simulink model "robot_step"  (Simulink 7.4)
settings: Solver=FixedStepDiscrete  StartTime=0.0  StopTime=50  FixedStep=0.1  RelTol=1e-3
values from neighbouring files (symbols this model uses):
  Link1 = [pi/2, 0, pi/2, 0]    [robot_parameters.m]
  Link2 = [0, 0.404, pi/2, 0]    [robot_parameters.m]
  Link3 = [-pi/2, 0, 0, 0]    [robot_parameters.m]
  Link4 = [pi/2, 0.025, 0, 0.405]    [robot_parameters.m]
  Link5 = [pi/2, 0, pi/2, 0]    [robot_parameters.m]
  Link6 = [0, 0, pi/2, 0]    [robot_parameters.m]
  NoOfLinks = 6    [robot_parameters.m]
libraries: vrlib x3, simulink x2
settings Model: Creator=angelosanto  LastModifiedBy=indranilsaha  BufferReuse=off
settings OptimizationCC: BlockReduction=off  BooleanDataType=off  ConditionallyExecuteInputs=off  InlineParams=on  OptimizeBlockIOStorage=off  BufferReuse=off  ExpressionFolding=off  LocalBlockOutputs=off
settings RTWCC: GenCodeOnly=on  GenerateMakefile=off

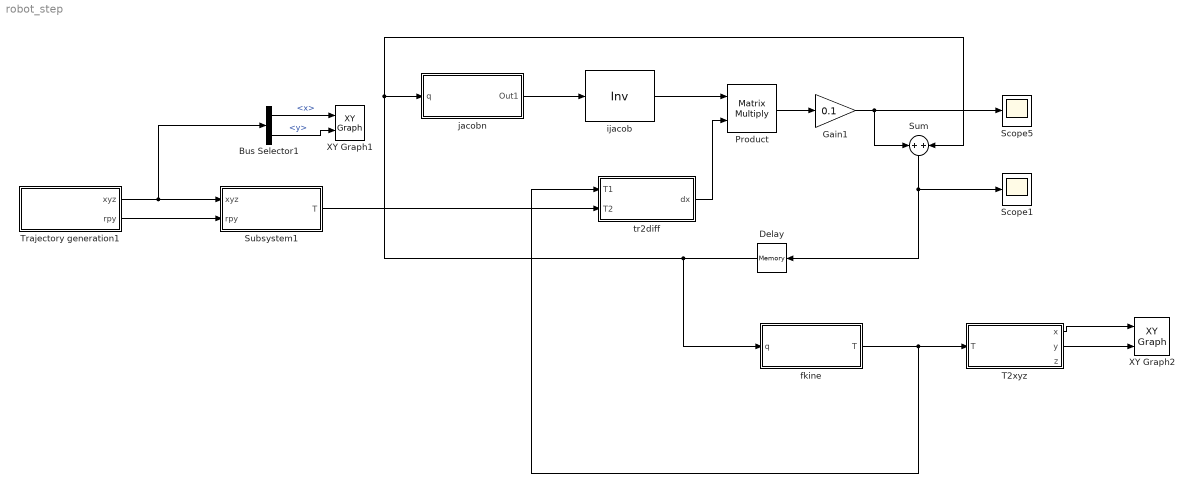
== system robot_step ==
  Bus Selector1 : BusSelector  OutputSignals=x,y
  Delay : Memory  X0=[pi/2; pi/2; 0; 0; pi/2; pi/2]  InheritSampleTime=on
  Gain1 : Gain  Gain=0.1  ParameterDataType=fixdt(1, 16)  ParameterScaling=2^0  OutDataType=fixdt(1, 16)  OutScaling=2^0
  Product : Product  Multiplication=Matrix(*)  OutDataType=sfix(16)  OutScaling=2^0  RndMeth=Zero
  Scope1 : Scope
      settings: YMin=-1  YMax=4
  Scope5 : Scope
      settings: YMin=-0.0003  YMax=0.00025  SaveName=ScopeData3
  Subsystem1 : Subsystem
  Sum : Sum  OutDataType=sfix(16)  OutScaling=2^0
  T2xyz : Subsystem
  Trajectory generation1 : Subsystem
  XY Graph1 : simulink/Sinks/XY Graph  SystemSampleTime=-1  xmin=-1.5  xmax=1.5  ymin=-1.5  ymax=1.5  st=-1
  XY Graph2 : simulink/Sinks/XY Graph  SystemSampleTime=-1  xmin=-1.5  xmax=1.5  ymin=-1.5  ymax=1.5  st=-1
  fkine : Subsystem  TreatAsAtomicUnit=on
  ijacob : Product  Inputs=/  Multiplication=Matrix(*)  OutDataType=fixdt(1, 16)  OutScaling=2^0  RndMeth=Zero
  jacobn : Subsystem  TreatAsAtomicUnit=on
  tr2diff : Subsystem
  wires:
  T2xyz/1(x) -> XY Graph2/1
  T2xyz/2(y) -> XY Graph2/2
  fkine/1(T) -> T2xyz/1(T), tr2diff/1(T1)
  jacobn/1(Out1) -> ijacob/1
  ijacob/1 -> Product/1
  tr2diff/1(dx) -> Product/2
  Sum/1 -> Delay/1, Scope1/1
  Delay/1 -> Sum/2, jacobn/1(q), fkine/1(q)
  Trajectory generation1/1(xyz) -> Subsystem1/1(xyz), Bus Selector1/1
  Trajectory generation1/2(rpy) -> Subsystem1/2(rpy)
  Bus Selector1/1 -> XY Graph1/1  "<x>"
  Bus Selector1/2 -> XY Graph1/2  "<y>"
  Subsystem1/1(T) -> tr2diff/2(T2)
  Product/1 -> Gain1/1
  Gain1/1 -> Scope5/1, Sum/1

== system robot_step/Subsystem1 ==
  xyz : Inport  OutDataType=fixdt(1, 16)  OutScaling=2^0
  rpy : Inport  Port=2  OutDataType=fixdt(1, 16)  OutScaling=2^0
  Bus Selector : BusSelector  OutputSignals=x,y,z
  Bus Selector1 : BusSelector  OutputSignals=roll,pitch,yaw
  Product : Product  Multiplication=Matrix(*)  OutDataType=fixdt(1, 16)  OutScaling=2^0  RndMeth=Zero
  rpy2T : Subsystem
  xyz2T : Subsystem
  T : Outport  OutDataType=fixdt(1, 16)  OutScaling=2^0
  wires:
  xyz/1 -> Bus Selector/1
  Bus Selector/1 -> xyz2T/1(x)  "<x>"
  Bus Selector/2 -> xyz2T/2(y)  "<y>"
  Bus Selector/3 -> xyz2T/3(z)  "<z>"
  xyz2T/1(T) -> Product/1
  Product/1 -> T/1
  rpy2T/1(T) -> Product/2
  rpy/1 -> Bus Selector1/1
  Bus Selector1/1 -> rpy2T/1(roll)  "<roll>"
  Bus Selector1/2 -> rpy2T/2(pitch)  "<pitch>"
  Bus Selector1/3 -> rpy2T/3(yaw)  "<yaw>"

== system robot_step/T2xyz ==
  T : Inport  OutDataType=fixdt(1, 16)  OutScaling=2^0
  Selector : Selector  NumberOfDimensions=2  InputPortWidth=3  IndexOptions=Index vector (dialog),Index vector (dialog)  Indices=1,4  OutputSizes=1,1
  Selector1 : Selector  NumberOfDimensions=2  InputPortWidth=3  IndexOptions=Index vector (dialog),Index vector (dialog)  Indices=2,4  OutputSizes=1,1
  Selector2 : Selector  NumberOfDimensions=2  InputPortWidth=3  IndexOptions=Index vector (dialog),Index vector (dialog)  Indices=3,4  OutputSizes=1,1
  x : Outport  OutDataType=fixdt(1, 16)  OutScaling=2^0
  y : Outport  Port=2  OutDataType=fixdt(1, 16)  OutScaling=2^0
  z : Outport  Port=3  OutDataType=fixdt(1, 16)  OutScaling=2^0
  wires:
  Selector/1 -> x/1
  Selector1/1 -> y/1
  Selector2/1 -> z/1
  T/1 -> Selector/1, Selector2/1, Selector1/1

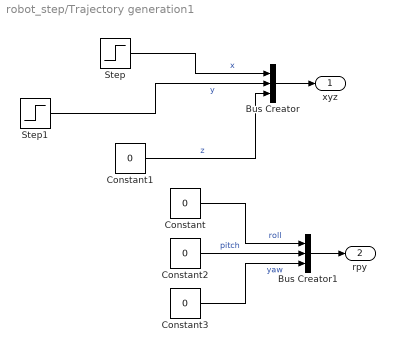
== system robot_step/Trajectory generation1 ==
  Bus Creator : BusCreator  Inputs=3
  Bus Creator1 : BusCreator  Inputs=3
  Constant : Constant  Value=0  VectorParams1D=off  OutDataType=fixdt(1, 16)  OutScaling=2^0
  Constant1 : Constant  Value=0
  Constant2 : Constant  Value=0  OutDataType=fixdt(1, 16)  OutScaling=2^0
  Constant3 : Constant  Value=0  OutDataType=fixdt(1, 16)  OutScaling=2^0
  Step : Step  After=0.3  SampleTime=0
  Step1 : Step  After=0.3  SampleTime=0
  xyz : Outport  OutDataType=fixdt(1, 16)  OutScaling=2^0
  rpy : Outport  Port=2  OutDataType=fixdt(1, 16)  OutScaling=2^0
  wires:
  Constant1/1 -> Bus Creator/3  "z"
  Bus Creator/1 -> xyz/1
  Constant2/1 -> Bus Creator1/2  "pitch"
  Constant/1 -> Bus Creator1/1  "roll"
  Constant3/1 -> Bus Creator1/3  "yaw"
  Bus Creator1/1 -> rpy/1
  Step/1 -> Bus Creator/1  "x"
  Step1/1 -> Bus Creator/2  "y"

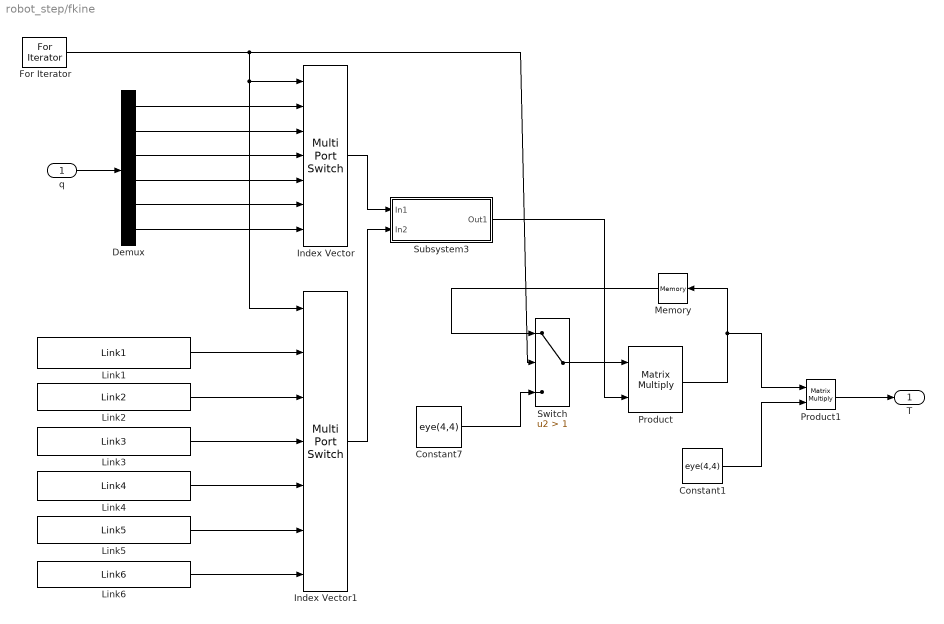
== system robot_step/fkine ==
  q : Inport  OutDataType=fixdt(1, 16)  OutScaling=2^0
  Constant1 : Constant  Value=eye(4,4)  OutDataType=fixdt(1, 16)  OutScaling=2^0
  Constant7 : Constant  Value=eye(4,4)  OutDataType=fixdt(1, 16)  OutScaling=2^0
  Demux : Demux  Outputs=6
  For Iterator : ForIterator  IterationLimit=NoOfLinks
  Index Vector : MultiPortSwitch  Inputs=6  OutDataType=fixdt(1, 16)  OutScaling=2^0
  Index Vector1 : MultiPortSwitch  Inputs=6  OutDataType=fixdt(1, 16)  OutScaling=2^0
  Link1 : Constant  Value=Link1  OutDataType=fixdt(1, 16)  OutScaling=2^0
  Link2 : Constant  Value=Link2  OutDataType=fixdt(1, 16)  OutScaling=2^0
  Link3 : Constant  Value=Link3  OutDataType=fixdt(1, 16)  OutScaling=2^0
  Link4 : Constant  Value=Link4  OutDataType=fixdt(1, 16)  OutScaling=2^0
  Link5 : Constant  Value=Link5  OutDataType=fixdt(1, 16)  OutScaling=2^0
  Link6 : Constant  Value=Link6  OutDataType=fixdt(1, 16)  OutScaling=2^0
  Memory : Memory  X0=eye(4,4)  InheritSampleTime=on
  Product : Product  Multiplication=Matrix(*)  OutDataType=fixdt(1, 16)  OutScaling=2^0  RndMeth=Zero
  Product1 : Product  Multiplication=Matrix(*)  OutDataType=fixdt(1, 16)  OutScaling=2^0  RndMeth=Zero
  Subsystem3 : Subsystem
  Switch : Switch  Criteria=u2 > Threshold  Threshold=1  OutDataType=fixdt(1, 16)  OutScaling=2^0
  T : Outport  OutDataType=fixdt(1, 16)  OutScaling=2^0
  wires:
  Memory/1 -> Switch/1
  Switch/1 -> Product/1
  Subsystem3/1(Out1) -> Product/2
  Constant7/1 -> Switch/3
  Product/1 -> Product1/1, Memory/1
  Index Vector1/1 -> Subsystem3/2(In2)
  Index Vector/1 -> Subsystem3/1(In1)
  Demux/6 -> Index Vector/7
  Demux/5 -> Index Vector/6
  Demux/4 -> Index Vector/5
  Demux/3 -> Index Vector/4
  Demux/2 -> Index Vector/3
  Demux/1 -> Index Vector/2
  q/1 -> Demux/1
  Link6/1 -> Index Vector1/7
  Link5/1 -> Index Vector1/6
  Link4/1 -> Index Vector1/5
  Link3/1 -> Index Vector1/4
  Link2/1 -> Index Vector1/3
  Link1/1 -> Index Vector1/2
  For Iterator/1 -> Switch/2, Index Vector1/1, Index Vector/1
  Product1/1 -> T/1
  Constant1/1 -> Product1/2

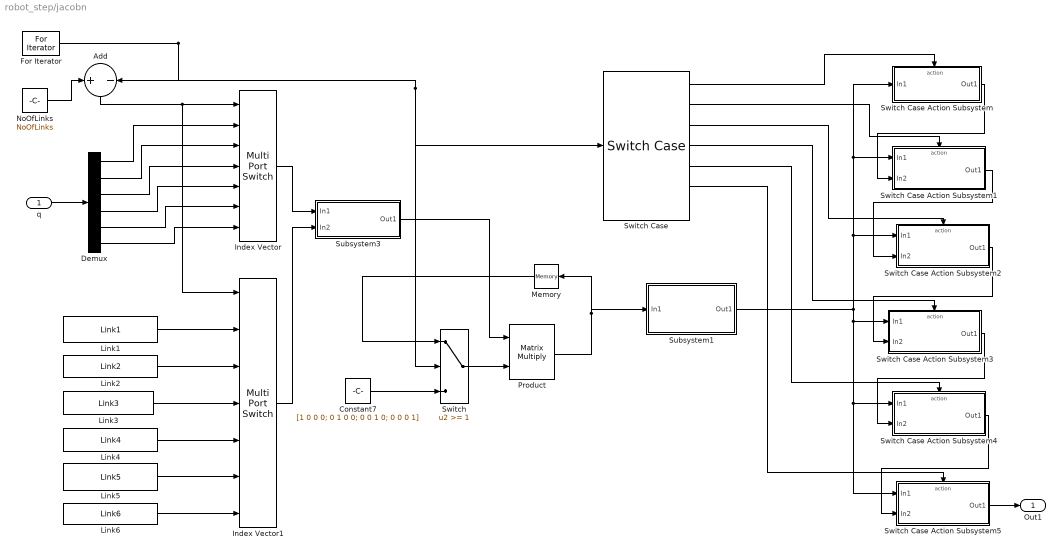
== system robot_step/jacobn ==
  q : Inport  OutDataType=fixdt(1, 16)  OutScaling=2^0
  Add : Sum  Inputs=+-  OutDataType=fixdt(1, 16)  OutScaling=2^-10
  Constant7 : Constant  Value=[1 0 0 0; 0 1 0 0; 0 0 1 0; 0 0 0 1]  OutDataType=fixdt(1, 16)  OutScaling=2^0
  Demux : Demux  Outputs=6
  For Iterator : ForIterator  IterationLimit=NoOfLinks
  Index Vector : MultiPortSwitch  Inputs=6  zeroidx=on  OutDataType=fixdt(1, 16)  OutScaling=2^0
  Index Vector1 : MultiPortSwitch  Inputs=6  zeroidx=on  OutDataType=fixdt(1, 16)  OutScaling=2^0
  Link1 : Constant  Value=Link1  OutDataType=fixdt(1, 16)  OutScaling=2^0
  Link2 : Constant  Value=Link2  OutDataType=fixdt(1, 16)  OutScaling=2^0
  Link3 : Constant  Value=Link3  OutDataType=fixdt(1, 16)  OutScaling=2^0
  Link4 : Constant  Value=Link4  OutDataType=fixdt(1, 16)  OutScaling=2^0
  Link5 : Constant  Value=Link5  OutDataType=fixdt(1, 16)  OutScaling=2^0
  Link6 : Constant  Value=Link6  OutDataType=fixdt(1, 16)  OutScaling=2^0
  Memory : Memory  X0=[1 0 0 0; 0 1 0 0; 0 0 1 0; 0 0 0 1]  InheritSampleTime=on
  NoOfLinks : Constant  Value=NoOfLinks  OutDataType=fixdt(1, 16)  OutScaling=2^0
  Product : Product  Multiplication=Matrix(*)  OutDataType=fixdt(1, 16)  OutScaling=2^0  RndMeth=Zero
  Subsystem1 : Subsystem
  Subsystem3 : Subsystem
  Switch : Switch  Threshold=1  OutDataType=fixdt(1, 16)  OutScaling=2^0
  Switch Case : SwitchCase  CaseConditions={1, 2, 3, 4, 5, 6}
  Switch Case Action Subsystem : Subsystem  TreatAsAtomicUnit=on
  Switch Case Action Subsystem1 : Subsystem  TreatAsAtomicUnit=on
  Switch Case Action Subsystem2 : Subsystem  TreatAsAtomicUnit=on
  Switch Case Action Subsystem3 : Subsystem  TreatAsAtomicUnit=on
  Switch Case Action Subsystem4 : Subsystem  TreatAsAtomicUnit=on
  Switch Case Action Subsystem5 : Subsystem  TreatAsAtomicUnit=on
  Out1 : Outport  OutDataType=fixdt(1, 16)  OutScaling=2^0
  wires:
  NoOfLinks/1 -> Add/1
  For Iterator/1 -> Add/2, Switch/2, Switch Case/1
  Add/1 -> Index Vector/1, Index Vector1/1
  Link1/1 -> Index Vector1/2
  Link2/1 -> Index Vector1/3
  Link3/1 -> Index Vector1/4
  Link4/1 -> Index Vector1/5
  Link5/1 -> Index Vector1/6
  Link6/1 -> Index Vector1/7
  q/1 -> Demux/1
  Demux/1 -> Index Vector/2
  Demux/2 -> Index Vector/3
  Demux/3 -> Index Vector/4
  Demux/4 -> Index Vector/5
  Demux/5 -> Index Vector/6
  Demux/6 -> Index Vector/7
  Index Vector/1 -> Subsystem3/1(In1)
  Index Vector1/1 -> Subsystem3/2(In2)
  Product/1 -> Memory/1, Subsystem1/1(In1)
  Constant7/1 -> Switch/3
  Subsystem3/1(Out1) -> Product/1
  Switch/1 -> Product/2
  Memory/1 -> Switch/1
  Subsystem1/1(Out1) -> Switch Case Action Subsystem/1(In1), Switch Case Action Subsystem1/1(In1), Switch Case Action Subsystem2/1(In1), Switch Case Action Subsystem5/1(In1), Switch Case Action Subsystem4/1(In1), Switch Case Action Subsystem3/1(In1)
  Switch Case/1 -> Switch Case Action Subsystem/Action
  Switch Case/2 -> Switch Case Action Subsystem1/Action
  Switch Case/3 -> Switch Case Action Subsystem2/Action
  Switch Case/4 -> Switch Case Action Subsystem3/Action
  Switch Case/5 -> Switch Case Action Subsystem4/Action
  Switch Case/6 -> Switch Case Action Subsystem5/Action
  Switch Case Action Subsystem5/1(Out1) -> Out1/1
  Switch Case Action Subsystem1/1(Out1) -> Switch Case Action Subsystem2/2(In2)
  Switch Case Action Subsystem/1(Out1) -> Switch Case Action Subsystem1/2(In2)
  Switch Case Action Subsystem2/1(Out1) -> Switch Case Action Subsystem3/2(In2)
  Switch Case Action Subsystem3/1(Out1) -> Switch Case Action Subsystem4/2(In2)
  Switch Case Action Subsystem4/1(Out1) -> Switch Case Action Subsystem5/2(In2)

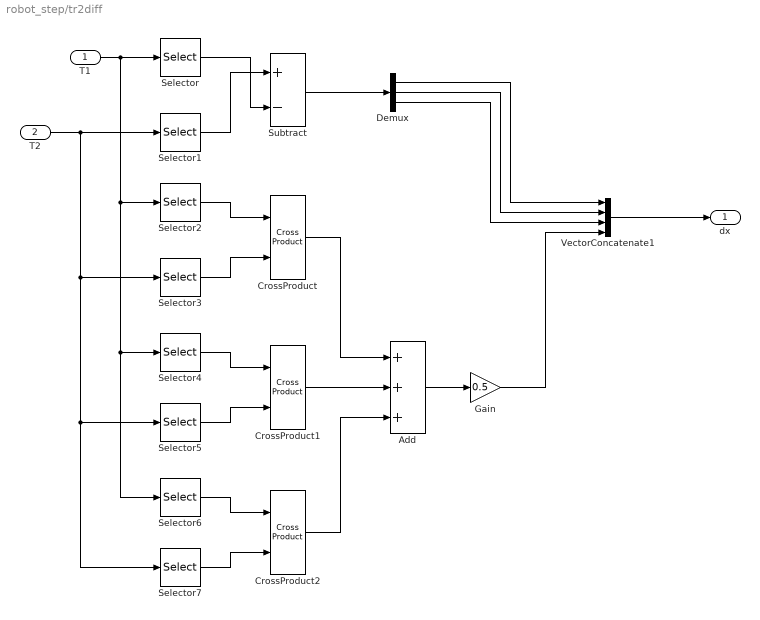
== system robot_step/tr2diff ==
  T1 : Inport  OutDataType=fixdt(1, 16)  OutScaling=2^0
  T2 : Inport  Port=2  OutDataType=fixdt(1, 16)  OutScaling=2^0
  Add : Sum  Inputs=+++  OutDataType=fixdt(1, 16)  OutScaling=2^-10
  CrossProduct : vrlib/Utilities/Cross Product  SystemSampleTime=-1
  CrossProduct1 : vrlib/Utilities/Cross Product  SystemSampleTime=-1
  CrossProduct2 : vrlib/Utilities/Cross Product  SystemSampleTime=-1
  Demux : Demux  Outputs=3
  Gain : Gain  Gain=0.5  ParameterDataType=fixdt(1, 16)  ParameterScaling=2^0  OutDataType=fixdt(1, 16)  OutScaling=2^0
  Selector : Selector  NumberOfDimensions=2  InputPortWidth=3  IndexOptions=Index vector (dialog),Index vector (dialog)  Indices=[1:3],4  OutputSizes=1,1
  Selector1 : Selector  NumberOfDimensions=2  InputPortWidth=3  IndexOptions=Index vector (dialog),Index vector (dialog)  Indices=[1:3],4  OutputSizes=1,1
  Selector2 : Selector  NumberOfDimensions=2  InputPortWidth=3  IndexOptions=Index vector (dialog),Index vector (dialog)  Indices=[1:3],1  OutputSizes=1,1
  Selector3 : Selector  NumberOfDimensions=2  InputPortWidth=3  IndexOptions=Index vector (dialog),Index vector (dialog)  Indices=[1:3],1  OutputSizes=1,1
  Selector4 : Selector  NumberOfDimensions=2  InputPortWidth=3  IndexOptions=Index vector (dialog),Index vector (dialog)  Indices=[1:3],2  OutputSizes=1,1
  Selector5 : Selector  NumberOfDimensions=2  InputPortWidth=3  IndexOptions=Index vector (dialog),Index vector (dialog)  Indices=[1:3],2  OutputSizes=1,1
  Selector6 : Selector  NumberOfDimensions=2  InputPortWidth=3  IndexOptions=Index vector (dialog),Index vector (dialog)  Indices=[1:3],3  OutputSizes=1,1
  Selector7 : Selector  NumberOfDimensions=2  InputPortWidth=3  IndexOptions=Index vector (dialog),Index vector (dialog)  Indices=[1:3],3  OutputSizes=1,1
  Subtract : Sum  Inputs=+-  OutDataType=fixdt(1, 16)  OutScaling=2^-10
  VectorConcatenate1 : Concatenate  NumInputs=4  Mode=Vector
  dx : Outport  OutDataType=fixdt(1, 16)  OutScaling=2^0
  wires:
  T1/1 -> Selector/1, Selector2/1, Selector6/1, Selector4/1
  T2/1 -> Selector1/1, Selector7/1, Selector5/1, Selector3/1
  Selector1/1 -> Subtract/1
  Selector/1 -> Subtract/2
  Selector2/1 -> CrossProduct/1
  Selector3/1 -> CrossProduct/2
  Selector4/1 -> CrossProduct1/1
  Selector5/1 -> CrossProduct1/2
  Selector6/1 -> CrossProduct2/1
  Selector7/1 -> CrossProduct2/2
  CrossProduct/1 -> Add/1
  CrossProduct1/1 -> Add/2
  CrossProduct2/1 -> Add/3
  Add/1 -> Gain/1
  VectorConcatenate1/1 -> dx/1
  Subtract/1 -> Demux/1
  Demux/1 -> VectorConcatenate1/1
  Demux/2 -> VectorConcatenate1/2
  Demux/3 -> VectorConcatenate1/3
  Gain/1 -> VectorConcatenate1/4

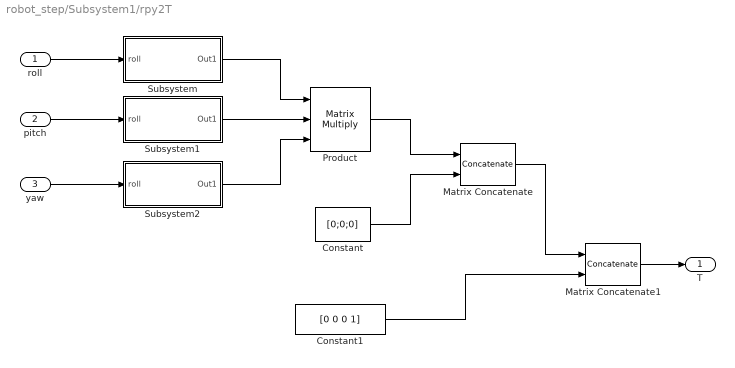
== system robot_step/Subsystem1/rpy2T ==
  roll : Inport  OutDataType=fixdt(1, 16)  OutScaling=2^0
  pitch : Inport  Port=2  OutDataType=fixdt(1, 16)  OutScaling=2^0
  yaw : Inport  Port=3  OutDataType=fixdt(1, 16)  OutScaling=2^0
  Constant : Constant  Value=[0;0;0]  OutDataType=fixdt(1, 16)  OutScaling=2^0
  Constant1 : Constant  Value=[0 0 0 1]  VectorParams1D=off  OutDataType=fixdt(1, 16)  OutScaling=2^0
  Matrix Concatenate : Concatenate  Mode=Multidimensional array  ConcatenateDimension=2
  Matrix Concatenate1 : Concatenate  Mode=Multidimensional array
  Product : Product  Inputs=3  Multiplication=Matrix(*)  OutDataType=fixdt(1, 16)  OutScaling=2^0  RndMeth=Zero
  Subsystem : Subsystem
  Subsystem1 : Subsystem
  Subsystem2 : Subsystem
  T : Outport  OutDataType=fixdt(1, 16)  OutScaling=2^0
  wires:
  roll/1 -> Subsystem/1(roll)
  pitch/1 -> Subsystem1/1(roll)
  yaw/1 -> Subsystem2/1(roll)
  Subsystem/1(Out1) -> Product/1
  Subsystem1/1(Out1) -> Product/2
  Subsystem2/1(Out1) -> Product/3
  Product/1 -> Matrix Concatenate/1
  Constant/1 -> Matrix Concatenate/2
  Matrix Concatenate/1 -> Matrix Concatenate1/1
  Constant1/1 -> Matrix Concatenate1/2
  Matrix Concatenate1/1 -> T/1

== system robot_step/Subsystem1/xyz2T ==
  x : Inport  OutDataType=fixdt(1, 16)  OutScaling=2^0
  y : Inport  Port=2  OutDataType=fixdt(1, 16)  OutScaling=2^0
  z : Inport  Port=3  OutDataType=fixdt(1, 16)  OutScaling=2^0
  Constant : Constant  Value=eye(3)  OutDataType=fixdt(1, 16)  OutScaling=2^0
  Constant1 : Constant  Value=[0 0 0 1]  VectorParams1D=off  OutDataType=fixdt(1, 16)  OutScaling=2^0
  Matrix Concatenate : Concatenate  Mode=Multidimensional array  ConcatenateDimension=2
  Matrix Concatenate1 : Concatenate  Mode=Multidimensional array
  Vector Concatenate : Concatenate  NumInputs=3  Mode=Vector
  T : Outport  OutDataType=fixdt(1, 16)  OutScaling=2^0
  wires:
  x/1 -> Vector Concatenate/1
  y/1 -> Vector Concatenate/2
  z/1 -> Vector Concatenate/3
  Constant/1 -> Matrix Concatenate/1
  Vector Concatenate/1 -> Matrix Concatenate/2
  Matrix Concatenate/1 -> Matrix Concatenate1/1
  Constant1/1 -> Matrix Concatenate1/2
  Matrix Concatenate1/1 -> T/1

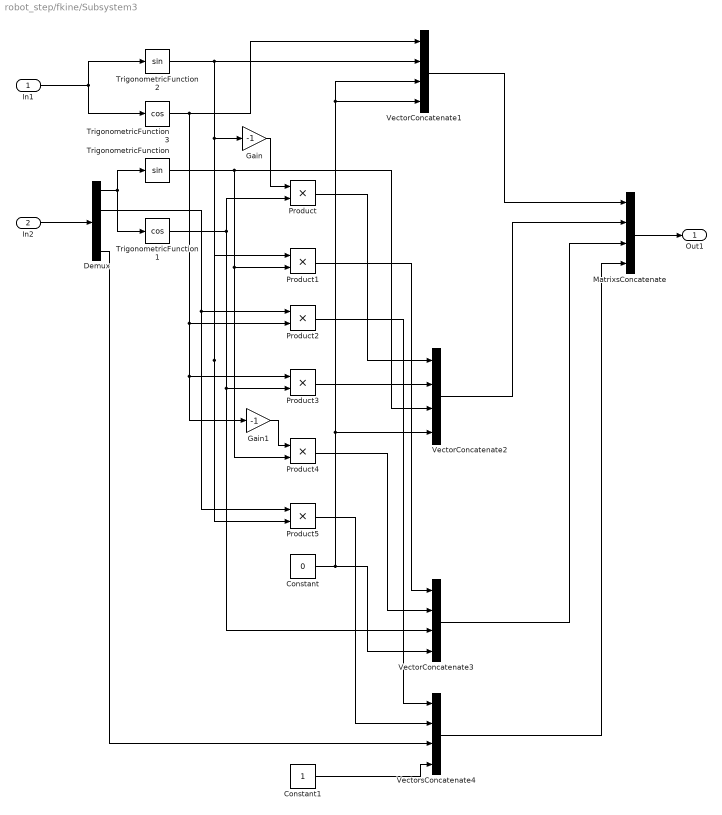
== system robot_step/fkine/Subsystem3 ==
  In1 : Inport  OutDataType=fixdt(1, 16)  OutScaling=2^0
  In2 : Inport  Port=2  OutDataType=fixdt(1, 16)  OutScaling=2^0
  Constant : Constant  Value=0  OutDataType=fixdt(1, 16)  OutScaling=2^0
  Constant1 : Constant  OutDataType=fixdt(1, 16)  OutScaling=2^0
  Demux : Demux
  Gain : Gain  Gain=-1  ParameterDataType=fixdt(1, 16)  ParameterScaling=2^0  OutDataType=fixdt(1, 16)  OutScaling=2^0
  Gain1 : Gain  Gain=-1  ParameterDataType=fixdt(1, 16)  ParameterScaling=2^0  OutDataType=fixdt(1, 16)  OutScaling=2^0
  MatrixsConcatenate : Concatenate  NumInputs=4  Mode=Multidimensional array  ConcatenateDimension=2
  Product{,1..5} (6 alike) : Product  OutDataType=fixdt(1, 16)  OutScaling=2^0  RndMeth=Zero
  TrigonometricFunction : Trigonometry
  TrigonometricFunction1 : Trigonometry  Operator=cos
  TrigonometricFunction2 : Trigonometry
  TrigonometricFunction3 : Trigonometry  Operator=cos
  VectorConcatenate1 : Concatenate  NumInputs=4  Mode=Vector  ConcatenateDimension=2
  VectorConcatenate2 : Concatenate  NumInputs=4  Mode=Vector  ConcatenateDimension=2
  VectorConcatenate3 : Concatenate  NumInputs=4  Mode=Vector  ConcatenateDimension=2
  VectorsConcatenate4 : Concatenate  NumInputs=4  Mode=Vector  ConcatenateDimension=2
  Out1 : Outport  OutDataType=fixdt(1, 16)  OutScaling=2^0
  wires:
  VectorsConcatenate4/1 -> MatrixsConcatenate/4
  VectorConcatenate3/1 -> MatrixsConcatenate/3
  VectorConcatenate2/1 -> MatrixsConcatenate/2
  VectorConcatenate1/1 -> MatrixsConcatenate/1
  MatrixsConcatenate/1 -> Out1/1
  Constant1/1 -> VectorsConcatenate4/4
  Constant/1 -> VectorConcatenate1/3, VectorConcatenate1/4, VectorConcatenate2/4, VectorConcatenate3/4
  Gain1/1 -> Product4/1
  Product3/1 -> VectorConcatenate2/2
  Demux/2 -> Product5/1, Product2/1
  TrigonometricFunction/1 -> Product1/2, Product4/2, VectorConcatenate2/3
  TrigonometricFunction3/1 -> VectorConcatenate1/1, Gain1/1, Product3/1, Product2/2
  TrigonometricFunction1/1 -> VectorConcatenate3/3, Product3/2, Product/2
  Gain/1 -> Product/1
  TrigonometricFunction2/1 -> Product1/1, Product5/2, Gain/1, VectorConcatenate1/2
  Demux/1 -> TrigonometricFunction1/1, TrigonometricFunction/1
  In1/1 -> TrigonometricFunction3/1, TrigonometricFunction2/1
  In2/1 -> Demux/1
  Product/1 -> VectorConcatenate2/1
  Product4/1 -> VectorConcatenate3/2
  Product1/1 -> VectorConcatenate3/1
  Product2/1 -> VectorsConcatenate4/1
  Product5/1 -> VectorsConcatenate4/2
  Demux/4 -> VectorsConcatenate4/3

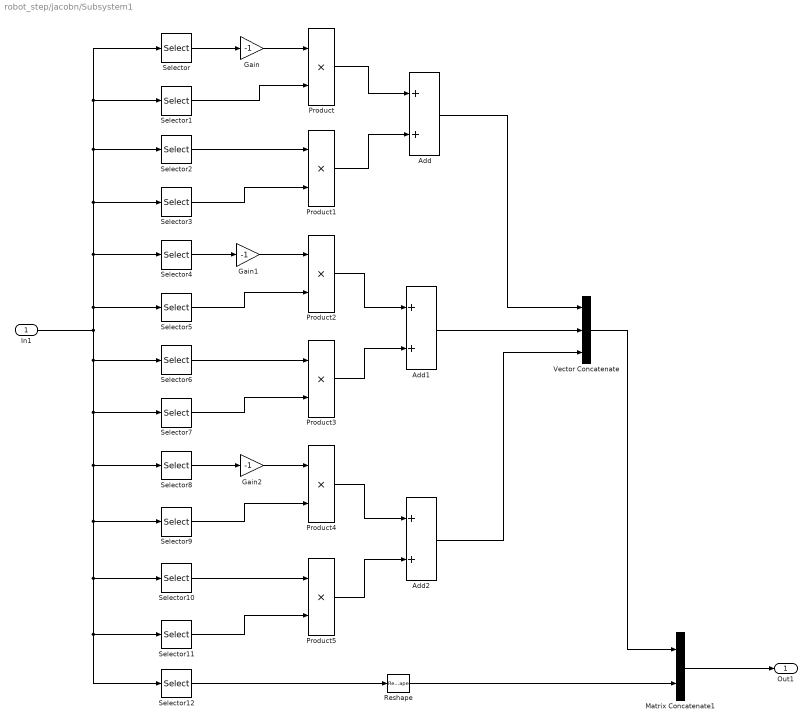
== system robot_step/jacobn/Subsystem1 ==
  In1 : Inport
  Add : Sum  OutDataType=fixdt(1, 16)  OutScaling=2^-10
  Add1 : Sum  OutDataType=fixdt(1, 16)  OutScaling=2^-10
  Add2 : Sum  OutDataType=fixdt(1, 16)  OutScaling=2^-10
  Gain : Gain  Gain=-1  ParameterDataType=fixdt(1, 16)  ParameterScaling=2^0  OutDataType=fixdt(1, 16)  OutScaling=2^0
  Gain1 : Gain  Gain=-1  ParameterDataType=fixdt(1, 16)  ParameterScaling=2^0  OutDataType=fixdt(1, 16)  OutScaling=2^0
  Gain2 : Gain  Gain=-1  ParameterDataType=fixdt(1, 16)  ParameterScaling=2^0  OutDataType=fixdt(1, 16)  OutScaling=2^0
  Matrix Concatenate1 : Concatenate  Mode=Multidimensional array
  Product{,1..5} (6 alike) : Product  OutDataType=fixdt(1, 16)  OutScaling=2^0  RndMeth=Zero
  Reshape : Reshape  OutputDimensionality=Customize  OutputDimensions=[3,1]
  Selector : Selector  NumberOfDimensions=2  InputPortWidth=3  IndexOptions=Index vector (dialog),Index vector (dialog)  Indices=1,1  OutputSizes=1,1
  Selector1 : Selector  NumberOfDimensions=2  InputPortWidth=3  IndexOptions=Index vector (dialog),Index vector (dialog)  Indices=2,4  OutputSizes=1,1
  Selector10 : Selector  NumberOfDimensions=2  InputPortWidth=3  IndexOptions=Index vector (dialog),Index vector (dialog)  Indices=2,3  OutputSizes=1,1
  Selector11 : Selector  NumberOfDimensions=2  InputPortWidth=3  IndexOptions=Index vector (dialog),Index vector (dialog)  Indices=1,4  OutputSizes=1,1
  Selector12 : Selector  NumberOfDimensions=2  InputPortWidth=3  IndexOptions=Index vector (dialog),Index vector (dialog)  Indices=3,[1:3]  OutputSizes=1,1
  Selector2 : Selector  NumberOfDimensions=2  InputPortWidth=3  IndexOptions=Index vector (dialog),Index vector (dialog)  Indices=2,1  OutputSizes=1,1
  Selector3 : Selector  NumberOfDimensions=2  InputPortWidth=3  IndexOptions=Index vector (dialog),Index vector (dialog)  Indices=1,4  OutputSizes=1,1
  Selector4 : Selector  NumberOfDimensions=2  InputPortWidth=3  IndexOptions=Index vector (dialog),Index vector (dialog)  Indices=1,2  OutputSizes=1,1
  Selector5 : Selector  NumberOfDimensions=2  InputPortWidth=3  IndexOptions=Index vector (dialog),Index vector (dialog)  Indices=2,4  OutputSizes=1,1
  Selector6 : Selector  NumberOfDimensions=2  InputPortWidth=3  IndexOptions=Index vector (dialog),Index vector (dialog)  Indices=2,2  OutputSizes=1,1
  Selector7 : Selector  NumberOfDimensions=2  InputPortWidth=3  IndexOptions=Index vector (dialog),Index vector (dialog)  Indices=1,4  OutputSizes=1,1
  Selector8 : Selector  NumberOfDimensions=2  InputPortWidth=3  IndexOptions=Index vector (dialog),Index vector (dialog)  Indices=1,3  OutputSizes=1,1
  Selector9 : Selector  NumberOfDimensions=2  InputPortWidth=3  IndexOptions=Index vector (dialog),Index vector (dialog)  Indices=2,4  OutputSizes=1,1
  Vector Concatenate : Concatenate  NumInputs=3  Mode=Vector
  Out1 : Outport
  wires:
  Selector/1 -> Gain/1
  In1/1 -> Selector/1, Selector1/1, Selector2/1, Selector3/1, Selector4/1, Selector5/1, Selector10/1, Selector11/1, Selector12/1, Selector9/1, Selector8/1, Selector7/1, Selector6/1
  Gain/1 -> Product/1
  Selector1/1 -> Product/2
  Selector2/1 -> Product1/1
  Selector3/1 -> Product1/2
  Selector4/1 -> Gain1/1
  Gain1/1 -> Product2/1
  Selector5/1 -> Product2/2
  Selector6/1 -> Product3/1
  Selector7/1 -> Product3/2
  Selector8/1 -> Gain2/1
  Gain2/1 -> Product4/1
  Selector9/1 -> Product4/2
  Selector10/1 -> Product5/1
  Selector11/1 -> Product5/2
  Product/1 -> Add/1
  Product1/1 -> Add/2
  Product2/1 -> Add1/1
  Product3/1 -> Add1/2
  Product4/1 -> Add2/1
  Product5/1 -> Add2/2
  Add/1 -> Vector Concatenate/1
  Add1/1 -> Vector Concatenate/2
  Add2/1 -> Vector Concatenate/3
  Vector Concatenate/1 -> Matrix Concatenate1/1
  Selector12/1 -> Reshape/1
  Matrix Concatenate1/1 -> Out1/1
  Reshape/1 -> Matrix Concatenate1/2

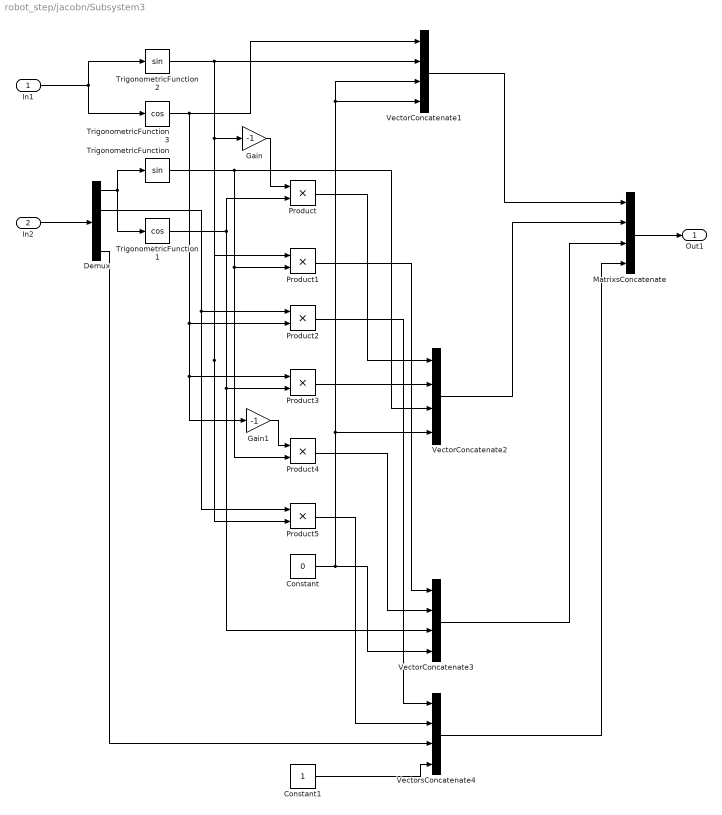
== system robot_step/jacobn/Subsystem3 ==
  In1 : Inport  OutDataType=fixdt(1, 16)  OutScaling=2^0
  In2 : Inport  Port=2  OutDataType=fixdt(1, 16)  OutScaling=2^0
  Constant : Constant  Value=0  OutDataType=fixdt(1, 16)  OutScaling=2^0
  Constant1 : Constant  OutDataType=fixdt(1, 16)  OutScaling=2^0
  Demux : Demux
  Gain : Gain  Gain=-1  ParameterDataType=fixdt(1, 16)  ParameterScaling=2^0  OutDataType=fixdt(1, 16)  OutScaling=2^0
  Gain1 : Gain  Gain=-1  ParameterDataType=fixdt(1, 16)  ParameterScaling=2^0  OutDataType=fixdt(1, 16)  OutScaling=2^0
  MatrixsConcatenate : Concatenate  NumInputs=4  Mode=Multidimensional array  ConcatenateDimension=2
  Product{,1..5} (6 alike) : Product  OutDataType=fixdt(1, 16)  OutScaling=2^0  RndMeth=Zero
  TrigonometricFunction : Trigonometry
  TrigonometricFunction1 : Trigonometry  Operator=cos
  TrigonometricFunction2 : Trigonometry
  TrigonometricFunction3 : Trigonometry  Operator=cos
  VectorConcatenate1 : Concatenate  NumInputs=4  Mode=Vector  ConcatenateDimension=2
  VectorConcatenate2 : Concatenate  NumInputs=4  Mode=Vector  ConcatenateDimension=2
  VectorConcatenate3 : Concatenate  NumInputs=4  Mode=Vector  ConcatenateDimension=2
  VectorsConcatenate4 : Concatenate  NumInputs=4  Mode=Vector  ConcatenateDimension=2
  Out1 : Outport  OutDataType=fixdt(1, 16)  OutScaling=2^0
  wires:
  VectorsConcatenate4/1 -> MatrixsConcatenate/4
  VectorConcatenate3/1 -> MatrixsConcatenate/3
  VectorConcatenate2/1 -> MatrixsConcatenate/2
  VectorConcatenate1/1 -> MatrixsConcatenate/1
  MatrixsConcatenate/1 -> Out1/1
  Constant1/1 -> VectorsConcatenate4/4
  Constant/1 -> VectorConcatenate1/3, VectorConcatenate1/4, VectorConcatenate2/4, VectorConcatenate3/4
  Gain1/1 -> Product4/1
  Product3/1 -> VectorConcatenate2/2
  Demux/2 -> Product5/1, Product2/1
  TrigonometricFunction/1 -> Product1/2, Product4/2, VectorConcatenate2/3
  TrigonometricFunction3/1 -> VectorConcatenate1/1, Gain1/1, Product3/1, Product2/2
  TrigonometricFunction1/1 -> VectorConcatenate3/3, Product3/2, Product/2
  Gain/1 -> Product/1
  TrigonometricFunction2/1 -> Product1/1, Product5/2, Gain/1, VectorConcatenate1/2
  Demux/1 -> TrigonometricFunction1/1, TrigonometricFunction/1
  In1/1 -> TrigonometricFunction3/1, TrigonometricFunction2/1
  In2/1 -> Demux/1
  Product/1 -> VectorConcatenate2/1
  Product4/1 -> VectorConcatenate3/2
  Product1/1 -> VectorConcatenate3/1
  Product2/1 -> VectorsConcatenate4/1
  Product5/1 -> VectorsConcatenate4/2
  Demux/4 -> VectorsConcatenate4/3

== system robot_step/jacobn/Switch Case Action Subsystem ==
  In1 : Inport  OutDataType=fixdt(1, 16)  OutScaling=2^0
  Action Port : ActionPort  ActionType=case
  Matrix Concatenate : Concatenate  NumInputs=1  Mode=Multidimensional array  ConcatenateDimension=2
  Out1 : Outport  OutDataType=fixdt(1, 16)  OutScaling=2^0
  wires:
  In1/1 -> Matrix Concatenate/1
  Matrix Concatenate/1 -> Out1/1

== system robot_step/jacobn/Switch Case Action Subsystem1 ==
  In1 : Inport  OutDataType=fixdt(1, 16)  OutScaling=2^0
  In2 : Inport  Port=2  OutDataType=fixdt(1, 16)  OutScaling=2^0
  Action Port : ActionPort  ActionType=case
  Matrix Concatenate : Concatenate  Mode=Multidimensional array  ConcatenateDimension=2
  Out1 : Outport  OutDataType=fixdt(1, 16)  OutScaling=2^0
  wires:
  In1/1 -> Matrix Concatenate/1
  In2/1 -> Matrix Concatenate/2
  Matrix Concatenate/1 -> Out1/1

== system robot_step/jacobn/Switch Case Action Subsystem2 ==
  In1 : Inport  OutDataType=fixdt(1, 16)  OutScaling=2^0
  In2 : Inport  Port=2  OutDataType=fixdt(1, 16)  OutScaling=2^0
  Action Port : ActionPort  ActionType=case
  Matrix Concatenate : Concatenate  Mode=Multidimensional array  ConcatenateDimension=2
  Out1 : Outport  OutDataType=fixdt(1, 16)  OutScaling=2^0
  wires:
  Matrix Concatenate/1 -> Out1/1
  In2/1 -> Matrix Concatenate/2
  In1/1 -> Matrix Concatenate/1

== system robot_step/jacobn/Switch Case Action Subsystem3 ==
  In1 : Inport  OutDataType=fixdt(1, 16)  OutScaling=2^0
  In2 : Inport  Port=2  OutDataType=fixdt(1, 16)  OutScaling=2^0
  Action Port : ActionPort  ActionType=case
  Matrix Concatenate : Concatenate  Mode=Multidimensional array  ConcatenateDimension=2
  Out1 : Outport  OutDataType=fixdt(1, 16)  OutScaling=2^0
  wires:
  In1/1 -> Matrix Concatenate/1
  In2/1 -> Matrix Concatenate/2
  Matrix Concatenate/1 -> Out1/1

== system robot_step/jacobn/Switch Case Action Subsystem4 ==
  In1 : Inport  OutDataType=fixdt(1, 16)  OutScaling=2^0
  In2 : Inport  Port=2  OutDataType=fixdt(1, 16)  OutScaling=2^0
  Action Port : ActionPort  ActionType=case
  Matrix Concatenate : Concatenate  Mode=Multidimensional array  ConcatenateDimension=2
  Out1 : Outport  OutDataType=fixdt(1, 16)  OutScaling=2^0
  wires:
  Matrix Concatenate/1 -> Out1/1
  In2/1 -> Matrix Concatenate/2
  In1/1 -> Matrix Concatenate/1

== system robot_step/jacobn/Switch Case Action Subsystem5 ==
  In1 : Inport  OutDataType=fixdt(1, 16)  OutScaling=2^0
  In2 : Inport  Port=2  OutDataType=fixdt(1, 16)  OutScaling=2^0
  Action Port : ActionPort  ActionType=case
  Matrix Concatenate : Concatenate  Mode=Multidimensional array  ConcatenateDimension=2
  Out1 : Outport  OutDataType=fixdt(1, 16)  OutScaling=2^0
  wires:
  In1/1 -> Matrix Concatenate/1
  In2/1 -> Matrix Concatenate/2
  Matrix Concatenate/1 -> Out1/1

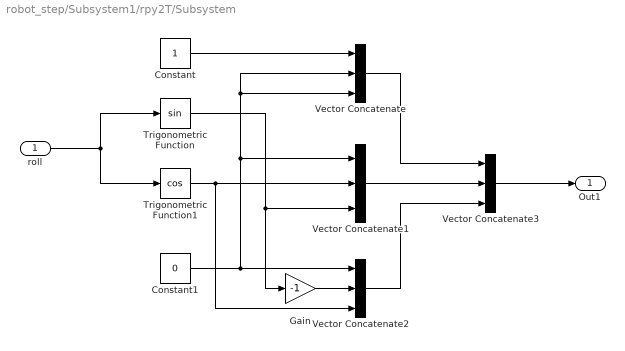
== system robot_step/Subsystem1/rpy2T/Subsystem ==
  roll : Inport  OutDataType=fixdt(1, 16)  OutScaling=2^0
  Constant : Constant  OutDataType=fixdt(1, 16)  OutScaling=2^0
  Constant1 : Constant  Value=0  OutDataType=fixdt(1, 16)  OutScaling=2^0
  Gain : Gain  Gain=-1  ParameterDataType=fixdt(1, 16)  ParameterScaling=2^0  OutDataType=fixdt(1, 16)  OutScaling=2^0
  Trigonometric Function : Trigonometry
  Trigonometric Function1 : Trigonometry  Operator=cos
  Vector Concatenate : Concatenate  NumInputs=3  Mode=Vector
  Vector Concatenate1 : Concatenate  NumInputs=3  Mode=Vector
  Vector Concatenate2 : Concatenate  NumInputs=3  Mode=Vector
  Vector Concatenate3 : Concatenate  NumInputs=3  Mode=Multidimensional array  ConcatenateDimension=2
  Out1 : Outport  OutDataType=fixdt(1, 16)  OutScaling=2^0
  wires:
  roll/1 -> Trigonometric Function/1, Trigonometric Function1/1
  Constant/1 -> Vector Concatenate/1
  Trigonometric Function1/1 -> Vector Concatenate1/2, Vector Concatenate2/3
  Trigonometric Function/1 -> Gain/1, Vector Concatenate1/3
  Vector Concatenate/1 -> Vector Concatenate3/1
  Vector Concatenate1/1 -> Vector Concatenate3/2
  Vector Concatenate2/1 -> Vector Concatenate3/3
  Constant1/1 -> Vector Concatenate/2, Vector Concatenate/3, Vector Concatenate1/1, Vector Concatenate2/1
  Gain/1 -> Vector Concatenate2/2
  Vector Concatenate3/1 -> Out1/1

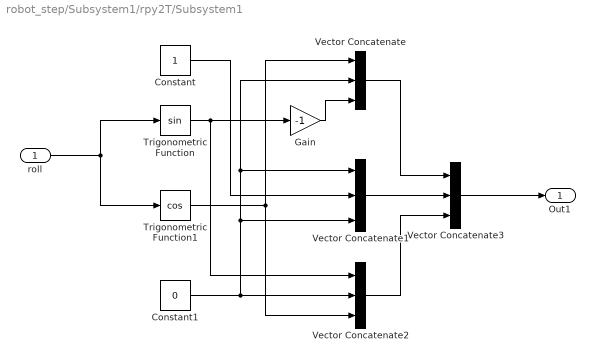
== system robot_step/Subsystem1/rpy2T/Subsystem1 ==
  roll : Inport  OutDataType=fixdt(1, 16)  OutScaling=2^0
  Constant : Constant  OutDataType=fixdt(1, 16)  OutScaling=2^0
  Constant1 : Constant  Value=0  OutDataType=fixdt(1, 16)  OutScaling=2^0
  Gain : Gain  Gain=-1  ParameterDataType=fixdt(1, 16)  ParameterScaling=2^0  OutDataType=fixdt(1, 16)  OutScaling=2^0
  Trigonometric Function : Trigonometry
  Trigonometric Function1 : Trigonometry  Operator=cos
  Vector Concatenate : Concatenate  NumInputs=3  Mode=Vector
  Vector Concatenate1 : Concatenate  NumInputs=3  Mode=Vector
  Vector Concatenate2 : Concatenate  NumInputs=3  Mode=Vector
  Vector Concatenate3 : Concatenate  NumInputs=3  Mode=Multidimensional array  ConcatenateDimension=2
  Out1 : Outport  OutDataType=fixdt(1, 16)  OutScaling=2^0
  wires:
  roll/1 -> Trigonometric Function/1, Trigonometric Function1/1
  Vector Concatenate/1 -> Vector Concatenate3/1
  Vector Concatenate1/1 -> Vector Concatenate3/2
  Vector Concatenate2/1 -> Vector Concatenate3/3
  Trigonometric Function1/1 -> Vector Concatenate/1, Vector Concatenate2/3
  Constant1/1 -> Vector Concatenate2/2, Vector Concatenate/2, Vector Concatenate1/1, Vector Concatenate1/3
  Trigonometric Function/1 -> Gain/1, Vector Concatenate2/1
  Constant/1 -> Vector Concatenate1/2
  Gain/1 -> Vector Concatenate/3
  Vector Concatenate3/1 -> Out1/1

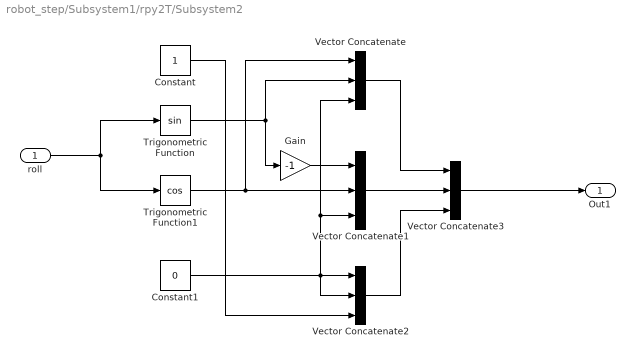
== system robot_step/Subsystem1/rpy2T/Subsystem2 ==
  roll : Inport  OutDataType=fixdt(1, 16)  OutScaling=2^0
  Constant : Constant  OutDataType=fixdt(1, 16)  OutScaling=2^0
  Constant1 : Constant  Value=0  OutDataType=fixdt(1, 16)  OutScaling=2^0
  Gain : Gain  Gain=-1  ParameterDataType=fixdt(1, 16)  ParameterScaling=2^0  OutDataType=fixdt(1, 16)  OutScaling=2^0
  Trigonometric Function : Trigonometry
  Trigonometric Function1 : Trigonometry  Operator=cos
  Vector Concatenate : Concatenate  NumInputs=3  Mode=Vector
  Vector Concatenate1 : Concatenate  NumInputs=3  Mode=Vector
  Vector Concatenate2 : Concatenate  NumInputs=3  Mode=Vector
  Vector Concatenate3 : Concatenate  NumInputs=3  Mode=Multidimensional array  ConcatenateDimension=2
  Out1 : Outport  OutDataType=fixdt(1, 16)  OutScaling=2^0
  wires:
  roll/1 -> Trigonometric Function/1, Trigonometric Function1/1
  Vector Concatenate/1 -> Vector Concatenate3/1
  Vector Concatenate1/1 -> Vector Concatenate3/2
  Vector Concatenate2/1 -> Vector Concatenate3/3
  Trigonometric Function1/1 -> Vector Concatenate/1, Vector Concatenate1/2
  Trigonometric Function/1 -> Vector Concatenate/2, Gain/1
  Constant1/1 -> Vector Concatenate/3, Vector Concatenate1/3, Vector Concatenate2/1, Vector Concatenate2/2
  Constant/1 -> Vector Concatenate2/3
  Gain/1 -> Vector Concatenate1/1
  Vector Concatenate3/1 -> Out1/1
